simulink library "sllib"  (R2018a)
settings: Solver=VariableStepAuto  StartTime=0.0  StopTime=10.0  RelTol=1e-3
undefined symbols (not defined in the file or in its folder): In2, Mask_inport
libraries: simulink x12, simulink_extras x2
settings Model: Creator=zhoutinglin  LastModifiedBy=zhoutinglin

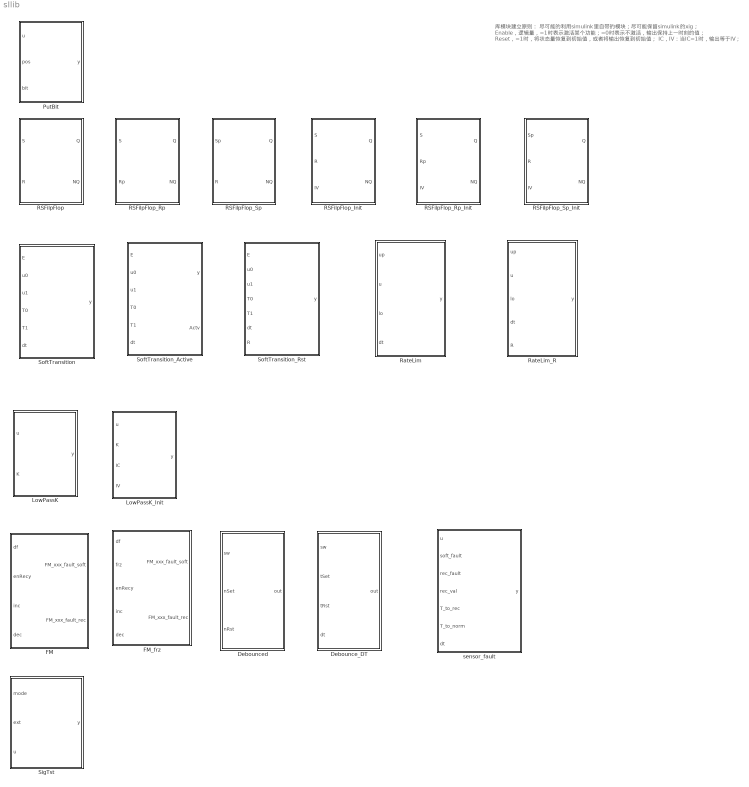
== system sllib ==
  note: 库模块建立原则：
      | 尽可能的利用simulink里自带的模块；尽可能保留simulink的xig；
      | Enable，逻辑量，=1时表示激活某个功能；=0时表示不激活，输出保持上一时刻的值；
      | Reset，=1时，将状态量恢复到初始值，或者将输出恢复到初始值；
      | IC，IV：当IC=1时，输出等于IV；
  Debounce_DT : Subsystem  mask(Debounce_DT){}
      mask help: 对一个开关形式的输入，当其状态改变时（从0变到1或者从1变到0），必须经过指定时间的确认之后再输出。
      mask Display:
      | color('blue');
      | plot([0.1,0.2,0.2,0.8,0.8,0.9],[0.26,0.26,0.46,0.46,0.26,0.26]);
      | plot([0.1,0.15,0.15,0.16,0.16,0.17,0.17,0.18,0.18,0.2,0.2,0.74,0.74,0.75,0.75,0.77,0.77,0.78,0.78,0.8,0.8,0.9],[0.55,0.55,0.75,0.75,0.55,0.55,0.75,0.75,0.55,0.55,0.75,0.75,0.55,0.55,0.75,0.75,0.55,0.55,0.75,0.75,0.55,0.55]);
  Debounced : Subsystem  mask(Debounced){}
      mask help: 对一个开关形式的输入，当其状态改变时（从0变到1或者从1变到0），必须经过指定次数的确认之后再输出。
      mask Display:
      | color('blue');
      | plot([0.1,0.2,0.2,0.8,0.8,0.9],[0.26,0.26,0.46,0.46,0.26,0.26]);
      | plot([0.1,0.15,0.15,0.16,0.16,0.17,0.17,0.18,0.18,0.2,0.2,0.74,0.74,0.75,0.75,0.77,0.77,0.78,0.78,0.8,0.8,0.9],[0.55,0.55,0.75,0.75,0.55,0.55,0.75,0.75,0.55,0.55,0.75,0.75,0.55,0.55,0.75,0.75,0.55,0.55,0.75,0.75,0.55,0.55]);
  FM : Subsystem  mask(FM){}
      mask help:
      | 输入df表示当前检测到的故障现象，等于1表示故障现象出现，等于0表示故障现象消失；
      | 输出soft故障等于输入df；
      | 输出rec故障等于soft故障经过Debounce后的状态。
  FM_frz : Subsystem  mask(FM_frz){}
      mask help:
      | 输入df表示当前检测到的故障现象，等于1表示故障现象出现，等于0表示故障现象消失；
      | 输出soft故障等于输入df；
      | 输出rec故障等于soft故障经过Debounce后的状态；
      | frz等于1后故障冻结，输出soft和rec的值不再变化，包括Debounce的计数器也不再变化。
  LowPassK : Subsystem  mask(LowPassK){}
      mask help: 低通滤波器
  LowPassK_Init : Subsystem  mask(LowPassK_Init){}
      mask help: 低通滤波器，带初始值。
  PutBit : Subsystem  mask(PutBit){}
      mask help: 给输入u在指定的位pos放入指定的值bit
  RSFilpFlop : Subsystem  mask(RSFlipFlop){}
      mask help: R和S都等于1时请参考真值表
  RSFilpFlop_Init : Subsystem  mask(RSFilpFlop_Init){}
      mask help:
      | R和S都等于1时请参考真值表;
      | 可以给Q赋初始值。
  RSFilpFlop_Rp : Subsystem  mask(RSFilpFlop_Rp){}
      mask help: R和S都等于1时的输出请参考真值表
  RSFilpFlop_Rp_Init : Subsystem  mask(RSFilpFlop_Rp_Init){}
      mask help:
      | R和S都等于1时请参考真值表;
      | 可以给Q赋初始值。
  RSFilpFlop_Sp : Subsystem  mask(RSFlipFlop_Sp){}
      mask help: R和S都等于1时的输出请参考真值表
  RSFilpFlop_Sp_Init : Subsystem  mask(RSFilpFlop_Sp_Init){}
      mask help:
      | R和S都等于1时请参考真值表;
      | 可以给Q赋初始值。
  RateLim : Subsystem  mask(RateLim){}
      mask help: 将输入信号u的变化速率限制在一定范围内。
  RateLim_R : Subsystem  mask(RateLim_R){}
      mask help: 将输入信号u的变化速率限制在一定范围内；当R置位时，输出y直接等于输入u。
  SigTst : Subsystem  mask(SigTst){}
      mask help:
      | 信号旁通功能，有3种模式：
      | mode=0时，直接输出u；
      | mode=1时，输出ext；
      | mode=2时，输出u+ext；
      mask Display:
      | color('white');
      | plot([0 0.01],[0 0.01]);
      | patch([0.65 0.67 0.67 0.65],[0.68 0.68 0.67 0.67]);
      | patch([0.65 0.67 0.67 0.65],[0.45 0.45 0.44 0.44]);
      | patch([0.65 0.67 0.67 0.65],[0.19 0.19 0.18 0.18]);
      | plot([0.18 0.65],[0.18 0.18]);
      | plot([0.18 0.65],[0.45 0.45]);
      | plot([0.24 0.4],[0.68 0.68]);
      | plot([0.57 0.65],[0.68 0.68]);
      | plot([0.4 0.57 0.57 0.4 0.4],[0.75 0.75 0.6 0.6 0.75]);
      | plot([0.49 0.49],[0.45 0.6]);
      | plot([0.45 0.52],[0.68 0.68]);
      | plot([0.49 0.49],[0.65 0.71]);
      | plot([0.24 0.24 0.26 0.26 0.24 0.24],[0.18 0.43 0.43 0.47 0.47 0.68]);
      | plot([0.25 0.85 0.85],[0.85 0.85 0.55]);
      | plot([0.7 0.8 0.95],[0.2 0.5 0.5]);
      | plot([0.83 0.85 0.88],[0.6 0.55 0.6])
  SoftTransition : Subsystem  mask(SoftTransition){}
      mask help: 当E改变时，输出缓慢过渡到u1或者u0.
  SoftTransition_Active : Subsystem  mask(SoftTransition_Active){}
      mask help:
      | 当E改变时，输出缓慢过渡到u1或者u0；
      | 输出Actv表示过渡是否已经结束。
  SoftTransition_Rst : Subsystem  mask(SoftTransition_Rst){}
      mask help:
      | 当E改变时，输出缓慢过渡到u1或者u0；
      | 当R置1时，直接输出目标值u1或者u0，不再过渡。
  sensor_fault : Subsystem  mask(sensor_fault){}
      mask help:
      | 当传感器无故障时，输出y直接等于输入u。
      | 当传感器有soft故障时，输出y等于其上一个时刻的值。
      | 当传感器故障被确认（rec）时，输出y过渡到rec_val；过渡时间为T_to_rec。
      | 当传感器从soft或rec状态恢复时，输出y经过时间T_to_norm过渡到u。

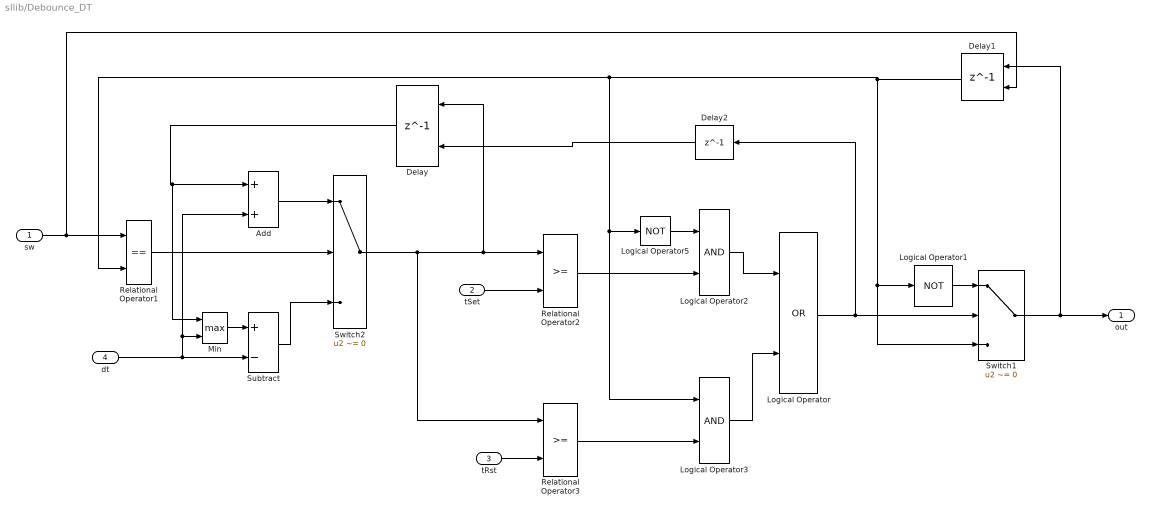
== system sllib/Debounce_DT ==
  sw : Inport  OutDataTypeStr=boolean
  tSet : Inport  Port=2
  tRst : Inport  Port=3
  dt : Inport  Port=4
  Add : Sum  SaturateOnIntegerOverflow=on  InputSameDT=on  OutDataTypeStr=Inherit: Same as first input
  Delay : Delay  DelayLength=1  ExternalReset=Rising
      settings: InputPortMap=u0,r5
  Delay1 : Delay  DelayLength=1  InitialConditionSource=Input port  InitialCondition=0
      settings: InputPortMap=u0,p4
  Delay2 : Delay  DelayLength=1  InitialCondition=0
  Logical Operator : Logic  Operator=OR  OutDataTypeStr=boolean
  Logical Operator1 : Logic  Operator=NOT  AllPortsSameDT=off  OutDataTypeStr=boolean
  Logical Operator2 : Logic  AllPortsSameDT=off  OutDataTypeStr=boolean
  Logical Operator3 : Logic  AllPortsSameDT=off  OutDataTypeStr=boolean
  Logical Operator5 : Logic  Operator=NOT  AllPortsSameDT=off  OutDataTypeStr=boolean
  Min : MinMax  Function=max  Inputs=2  ZeroCross=off  SaturateOnIntegerOverflow=on  InputSameDT=on
  Relational Operator1 : RelationalOperator  Operator===  OutDataTypeStr=boolean  ZeroCross=off  RndMeth=Simplest  InputSameDT=on
  Relational Operator2 : RelationalOperator  OutDataTypeStr=boolean  ZeroCross=off  RndMeth=Simplest  InputSameDT=on
  Relational Operator3 : RelationalOperator  OutDataTypeStr=boolean  ZeroCross=off  RndMeth=Simplest  InputSameDT=on
  Subtract : Sum  Inputs=+-  SaturateOnIntegerOverflow=on  InputSameDT=on
  Switch1 : Switch  Criteria=u2 ~= 0  ZeroCross=off
  Switch2 : Switch  Criteria=u2 ~= 0  ZeroCross=off  SaturateOnIntegerOverflow=on  InputSameDT=on
  out : Outport  OutDataTypeStr=boolean
  wires:
  Min/1 -> Subtract/1
  Delay2/1 -> Delay/2
  sw/1 -> Relational Operator1/1, Delay1/2
  Switch2/1 -> Relational Operator3/1, Delay/1, Relational Operator2/1
  Logical Operator/1 -> Switch1/2, Delay2/1
  Switch1/1 -> Delay1/1, out/1
  Delay/1 -> Add/1, Min/1
  Add/1 -> Switch2/1
  Relational Operator1/1 -> Switch2/2
  dt/1 -> Add/2, Min/2, Subtract/2
  Subtract/1 -> Switch2/3
  tSet/1 -> Relational Operator2/2
  tRst/1 -> Relational Operator3/2
  Logical Operator1/1 -> Switch1/1
  Relational Operator2/1 -> Logical Operator2/2
  Relational Operator3/1 -> Logical Operator3/2
  Delay1/1 -> Logical Operator3/1, Logical Operator5/1, Relational Operator1/2, Switch1/3, Logical Operator1/1
  Logical Operator2/1 -> Logical Operator/1
  Logical Operator3/1 -> Logical Operator/2
  Logical Operator5/1 -> Logical Operator2/1

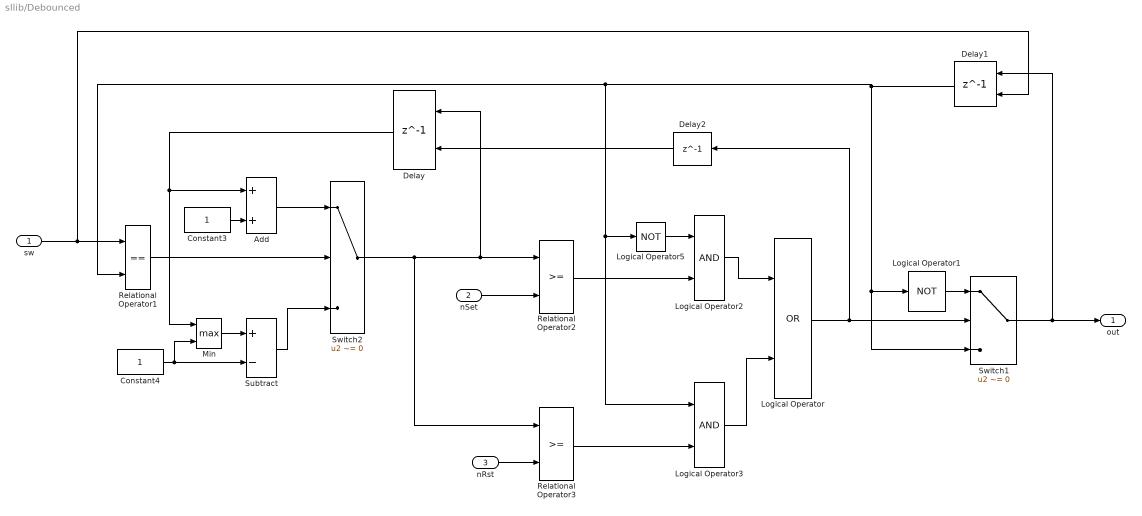
== system sllib/Debounced ==
  sw : Inport  OutDataTypeStr=boolean
  nSet : Inport  Port=2  OutDataTypeStr=uint16
  nRst : Inport  Port=3  OutDataTypeStr=uint16
  Add : Sum  SaturateOnIntegerOverflow=on  InputSameDT=on
  Constant3 : Constant  OutDataTypeStr=uint16
  Constant4 : Constant  OutDataTypeStr=uint16
  Delay : Delay  DelayLength=1  ExternalReset=Rising
      settings: InputPortMap=u0,r5
  Delay1 : Delay  DelayLength=1  InitialConditionSource=Input port
      settings: InputPortMap=u0,p4
  Delay2 : Delay  DelayLength=1  InitialCondition=0
  Logical Operator : Logic  Operator=OR  AllPortsSameDT=off  OutDataTypeStr=boolean
  Logical Operator1 : Logic  Operator=NOT  AllPortsSameDT=off  OutDataTypeStr=boolean
  Logical Operator2 : Logic  AllPortsSameDT=off  OutDataTypeStr=boolean
  Logical Operator3 : Logic  AllPortsSameDT=off  OutDataTypeStr=boolean
  Logical Operator5 : Logic  Operator=NOT  AllPortsSameDT=off  OutDataTypeStr=boolean
  Min : MinMax  Function=max  Inputs=2  ZeroCross=off  SaturateOnIntegerOverflow=on  InputSameDT=on
  Relational Operator1 : RelationalOperator  Operator===  OutDataTypeStr=boolean  ZeroCross=off  RndMeth=Simplest
  Relational Operator2 : RelationalOperator  OutDataTypeStr=boolean  ZeroCross=off  RndMeth=Simplest
  Relational Operator3 : RelationalOperator  OutDataTypeStr=boolean  ZeroCross=off  RndMeth=Simplest
  Subtract : Sum  Inputs=+-  SaturateOnIntegerOverflow=on  InputSameDT=on
  Switch1 : Switch  Criteria=u2 ~= 0  ZeroCross=off
  Switch2 : Switch  Criteria=u2 ~= 0  ZeroCross=off
  out : Outport  OutDataTypeStr=boolean
  wires:
  sw/1 -> Delay1/2, Relational Operator1/1
  Switch2/1 -> Relational Operator3/1, Delay/1, Relational Operator2/1
  Logical Operator/1 -> Switch1/2, Delay2/1
  Switch1/1 -> Delay1/1, out/1
  Delay/1 -> Min/1, Add/1
  Add/1 -> Switch2/1
  Relational Operator1/1 -> Switch2/2
  Constant3/1 -> Add/2
  Constant4/1 -> Subtract/2, Min/2
  Subtract/1 -> Switch2/3
  nSet/1 -> Relational Operator2/2
  nRst/1 -> Relational Operator3/2
  Logical Operator1/1 -> Switch1/1
  Relational Operator2/1 -> Logical Operator2/2
  Relational Operator3/1 -> Logical Operator3/2
  Delay1/1 -> Logical Operator3/1, Logical Operator5/1, Relational Operator1/2, Switch1/3, Logical Operator1/1
  Logical Operator2/1 -> Logical Operator/1
  Logical Operator3/1 -> Logical Operator/2
  Logical Operator5/1 -> Logical Operator2/1
  Delay2/1 -> Delay/2
  Min/1 -> Subtract/1

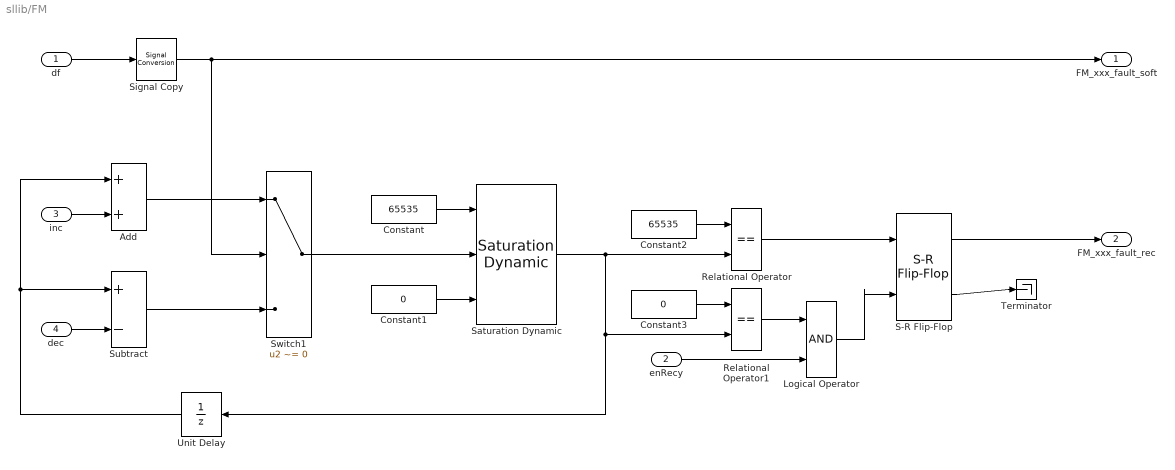
== system sllib/FM ==
  df : Inport  OutDataTypeStr=boolean
  enRecy : Inport  Port=2  OutDataTypeStr=boolean
  inc : Inport  LibraryBlock=Mask_inport/In2  Port=3  OutDataTypeStr=uint16
  dec : Inport  LibraryBlock=Mask_inport/In2  Port=4  OutDataTypeStr=uint16
  Add : Sum  SaturateOnIntegerOverflow=on  InputSameDT=on  OutDataTypeStr=Inherit: Same as first input
  Constant : Constant  Value=65535  OutDataTypeStr=uint16
  Constant1 : Constant  Value=0  OutDataTypeStr=uint16
  Constant2 : Constant  Value=65535  OutDataTypeStr=uint16
  Constant3 : Constant  Value=0  OutDataTypeStr=uint16
  Logical Operator : Logic  AllPortsSameDT=off  OutDataTypeStr=boolean
  Relational Operator : RelationalOperator  Operator===  OutDataTypeStr=boolean  ZeroCross=off  RndMeth=Simplest  InputSameDT=on
  Relational Operator1 : RelationalOperator  Operator===  OutDataTypeStr=boolean  ZeroCross=off  RndMeth=Simplest  InputSameDT=on
  S-R Flip-Flop : simulink_extras/Flip Flops/S-R Flip-Flop  initial_condition=0
      settings: AttributesFormatString=InitialValueQ=%<initial_condition>
  Saturation Dynamic : simulink/Discontinuities/Saturation Dynamic  OutMin=[]  OutMax=[]  OutDataTypeStr=Inherit: Same as second input  OutDataType=fixdt(1, 16)  OutScaling=2^-10  DoSatur=off
  Signal Copy : SignalConversion  OverrideOpt=off
  Subtract : Sum  Inputs=+-  SaturateOnIntegerOverflow=on  InputSameDT=on  OutDataTypeStr=Inherit: Same as first input
  Switch1 : Switch  Criteria=u2 ~= 0  ZeroCross=off  InputSameDT=on
  Terminator : Terminator
  Unit Delay : UnitDelay  SampleTime=-1
      settings: AttributesFormatString=InitialValue=%<InitialCondition>
  FM_xxx_fault_soft : Outport  OutDataTypeStr=boolean
  FM_xxx_fault_rec : Outport  Port=2  OutDataTypeStr=boolean
  wires:
  Signal Copy/1 -> FM_xxx_fault_soft/1, Switch1/2
  S-R Flip-Flop/1 -> FM_xxx_fault_rec/1
  S-R Flip-Flop/2 -> Terminator/1
  Logical Operator/1 -> S-R Flip-Flop/2
  Relational Operator/1 -> S-R Flip-Flop/1
  Relational Operator1/1 -> Logical Operator/1
  Constant3/1 -> Relational Operator1/1
  Saturation Dynamic/1 -> Relational Operator1/2, Unit Delay/1, Relational Operator/2
  Constant2/1 -> Relational Operator/1
  Constant1/1 -> Saturation Dynamic/3
  Constant/1 -> Saturation Dynamic/1
  Switch1/1 -> Saturation Dynamic/2
  Subtract/1 -> Switch1/3
  Add/1 -> Switch1/1
  Unit Delay/1 -> Add/1, Subtract/1
  inc/1 -> Add/2
  dec/1 -> Subtract/2
  enRecy/1 -> Logical Operator/2
  df/1 -> Signal Copy/1

== system sllib/FM_frz ==
  df : Inport  OutDataTypeStr=boolean
  frz : Inport  Port=2  OutDataTypeStr=boolean
  enRecy : Inport  Port=3  OutDataTypeStr=boolean
  inc : Inport  LibraryBlock=Mask_inport/In2  Port=4  OutDataTypeStr=uint16
  dec : Inport  LibraryBlock=Mask_inport/In2  Port=5  OutDataTypeStr=uint16
  rec : Subsystem
  soft : Subsystem
  FM_xxx_fault_soft : Outport  OutDataTypeStr=boolean
  FM_xxx_fault_rec : Outport  Port=2  OutDataTypeStr=boolean
  wires:
  inc/1 -> rec/4(inc)
  dec/1 -> rec/5(dec)
  soft/1(FM_xxx_fault_soft) -> FM_xxx_fault_soft/1
  rec/1(FM_xxx_fault_rec) -> FM_xxx_fault_rec/1
  df/1 -> rec/1(df), soft/1(df)
  frz/1 -> rec/2(frz), soft/2(frz)
  enRecy/1 -> rec/3(enRecy)

== system sllib/LowPassK ==
  u : Inport
  K : Inport  Port=2
  Delay : Delay  DelayLength=1  InitialConditionSource=Input port
      settings: InputPortMap=u0,p4
  Product : Product  RndMeth=Round  SaturateOnIntegerOverflow=on  OutDataTypeStr=Inherit: Same as first input
  Subtract1 : Sum  Inputs=+-  RndMeth=Round  SaturateOnIntegerOverflow=on  InputSameDT=on  OutDataTypeStr=Inherit: Same as first input
  Sum : Sum  Inputs=+|+  RndMeth=Round  SaturateOnIntegerOverflow=on  InputSameDT=on  OutDataTypeStr=Inherit: Same as first input
  y : Outport
  wires:
  u/1 -> Delay/2, Subtract1/1
  Delay/1 -> Sum/2, Subtract1/2
  Product/1 -> Sum/1
  Sum/1 -> Delay/1, y/1
  Subtract1/1 -> Product/1
  K/1 -> Product/2

== system sllib/LowPassK_Init ==
  u : Inport
  K : Inport  Port=2
  IC : Inport  Port=3  OutDataTypeStr=boolean
  IV : Inport  Port=4
  Delay : Delay  DelayLength=1  InitialConditionSource=Input port
      settings: InputPortMap=u0,p4
  Product : Product  RndMeth=Round  SaturateOnIntegerOverflow=on  OutDataTypeStr=Inherit: Same as first input
  Subtract1 : Sum  Inputs=+-  RndMeth=Round  SaturateOnIntegerOverflow=on  InputSameDT=on  OutDataTypeStr=Inherit: Same as first input
  Sum : Sum  Inputs=+|+  RndMeth=Round  SaturateOnIntegerOverflow=on  InputSameDT=on  OutDataTypeStr=Inherit: Same as first input
  Switch : Switch  Criteria=u2 ~= 0  RndMeth=Round  ZeroCross=off  InputSameDT=on
  y : Outport
  wires:
  Switch/1 -> Delay/1, y/1
  IC/1 -> Switch/2
  IV/1 -> Switch/1
  Subtract1/1 -> Product/1
  Delay/1 -> Sum/2, Subtract1/2
  u/1 -> Delay/2, Subtract1/1
  Sum/1 -> Switch/3
  Product/1 -> Sum/1
  K/1 -> Product/2

== system sllib/PutBit ==
  u : Inport
  pos : Inport  Port=2  OutDataTypeStr=uint8
  bit : Inport  Port=3  OutDataTypeStr=boolean
  Bitwise Operator : simulink/Logic and Bit Operations/Bitwise Operator  logicop=OR  UseBitMask=off  NumInputPorts=2  BitMask=bin2dec('11011001')  BitMaskRealWorld=Stored Integer
  Bitwise Operator1 : simulink/Logic and Bit Operations/Bitwise Operator  logicop=AND  UseBitMask=off  NumInputPorts=2  BitMask=bin2dec('11011001')  BitMaskRealWorld=Stored Integer
  Bitwise Operator2 : simulink/Logic and Bit Operations/Bitwise Operator  logicop=NOT  UseBitMask=off  BitMask=bin2dec('11011001')  BitMaskRealWorld=Stored Integer
  Constant2 : Constant  OutDataTypeStr=Inherit: Inherit via back propagation
  Data Type Duplicate : DataTypeDuplicate  NumInputPorts=3
  Shift Arithmetic : ArithShift  BitShiftNumberSource=Input port  BitShiftNumber=8  BitShiftDirection=Left
      settings: InputPortMap=u0,p1
  Switch : Switch  Criteria=u2 ~= 0  RndMeth=Round  ZeroCross=off  InputSameDT=on
  y : Outport
  wires:
  pos/1 -> Shift Arithmetic/2
  Constant2/1 -> Data Type Duplicate/2, Shift Arithmetic/1
  Shift Arithmetic/1 -> Bitwise Operator2/1, Bitwise Operator/2
  bit/1 -> Switch/2
  Bitwise Operator/1 -> Switch/1
  u/1 -> Data Type Duplicate/1, Bitwise Operator1/1, Bitwise Operator/1
  Bitwise Operator2/1 -> Bitwise Operator1/2
  Bitwise Operator1/1 -> Switch/3
  Switch/1 -> Data Type Duplicate/3, y/1

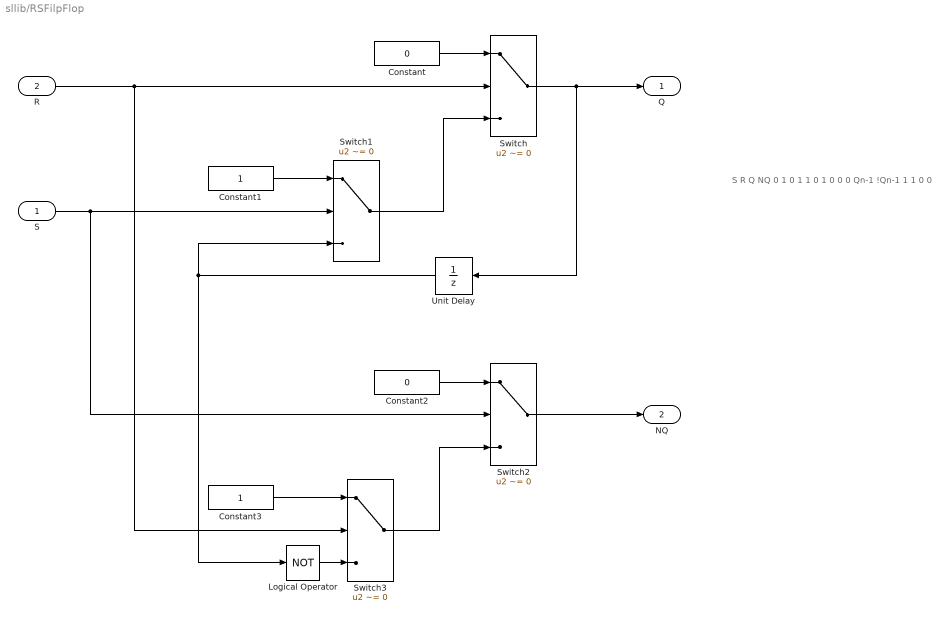
== system sllib/RSFilpFlop ==
  note: S
      | R
      | Q
      | NQ
      |
      | 0
      | 1
      | 0
      | 1
      |
      | 1
      | 0
      | 1
      | 0
      |
      | 0
      | 0
      | Qn-1
      | !Qn-1
      |
      | 1
      | 1
      | 0
      | 0
  S : Inport  OutDataTypeStr=boolean
  R : Inport  Port=2  OutDataTypeStr=boolean
  Constant : Constant  Value=0  OutDataTypeStr=boolean
  Constant1 : Constant  OutDataTypeStr=boolean
  Constant2 : Constant  Value=0  OutDataTypeStr=boolean
  Constant3 : Constant  OutDataTypeStr=boolean
  Logical Operator : Logic  Operator=NOT  AllPortsSameDT=off  OutDataTypeStr=boolean
  Switch{,1..3} (4 alike) : Switch  Criteria=u2 ~= 0  ZeroCross=off
  Unit Delay : UnitDelay  SampleTime=-1
      settings: AttributesFormatString=InitialValue=%<InitialCondition>
  Q : Outport  OutDataTypeStr=boolean
  NQ : Outport  Port=2  OutDataTypeStr=boolean
  wires:
  R/1 -> Switch3/2, Switch/2
  Constant/1 -> Switch/1
  Switch/1 -> Unit Delay/1, Q/1
  S/1 -> Switch2/2, Switch1/2
  Constant1/1 -> Switch1/1
  Switch1/1 -> Switch/3
  Unit Delay/1 -> Switch1/3, Logical Operator/1
  Switch2/1 -> NQ/1
  Constant2/1 -> Switch2/1
  Switch3/1 -> Switch2/3
  Constant3/1 -> Switch3/1
  Logical Operator/1 -> Switch3/3

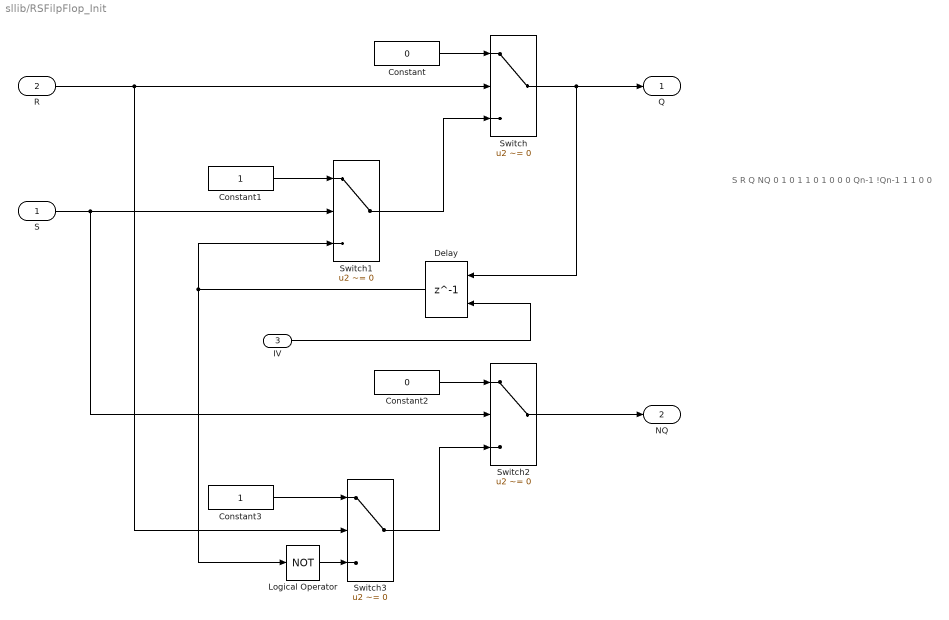
== system sllib/RSFilpFlop_Init ==
  note: S
      | R
      | Q
      | NQ
      |
      | 0
      | 1
      | 0
      | 1
      |
      | 1
      | 0
      | 1
      | 0
      |
      | 0
      | 0
      | Qn-1
      | !Qn-1
      |
      | 1
      | 1
      | 0
      | 0
  S : Inport  OutDataTypeStr=boolean
  R : Inport  Port=2  OutDataTypeStr=boolean
  IV : Inport  Port=3
  Constant : Constant  Value=0  OutDataTypeStr=boolean
  Constant1 : Constant  OutDataTypeStr=boolean
  Constant2 : Constant  Value=0  OutDataTypeStr=boolean
  Constant3 : Constant  OutDataTypeStr=boolean
  Delay : Delay  DelayLength=1  InitialConditionSource=Input port
      settings: InputPortMap=u0,p4
  Logical Operator : Logic  Operator=NOT  AllPortsSameDT=off  OutDataTypeStr=boolean
  Switch{,1..3} (4 alike) : Switch  Criteria=u2 ~= 0  ZeroCross=off
  Q : Outport  OutDataTypeStr=boolean
  NQ : Outport  Port=2  OutDataTypeStr=boolean
  wires:
  R/1 -> Switch3/2, Switch/2
  Constant/1 -> Switch/1
  Switch/1 -> Delay/1, Q/1
  S/1 -> Switch2/2, Switch1/2
  Constant1/1 -> Switch1/1
  Switch1/1 -> Switch/3
  Delay/1 -> Switch1/3, Logical Operator/1
  Switch2/1 -> NQ/1
  Constant2/1 -> Switch2/1
  Switch3/1 -> Switch2/3
  Constant3/1 -> Switch3/1
  Logical Operator/1 -> Switch3/3
  IV/1 -> Delay/2

== system sllib/RSFilpFlop_Rp ==
  note: S
      | R
      | Q
      | NQ
      |
      | 0
      | 1
      | 0
      | 1
      |
      | 1
      | 0
      | 1
      | 0
      |
      | 0
      | 0
      | Qn-1
      | !Qn-1
      |
      | 1
      | 1
      | 0
      | 1
  S : Inport  OutDataTypeStr=boolean
  Rp : Inport  Port=2  OutDataTypeStr=boolean
  Constant : Constant  Value=0  OutDataTypeStr=boolean
  Constant1 : Constant  OutDataTypeStr=boolean
  Logical Operator : Logic  Operator=NOT  AllPortsSameDT=off  OutDataTypeStr=boolean
  Switch : Switch  Criteria=u2 ~= 0  ZeroCross=off
  Switch1 : Switch  Criteria=u2 ~= 0  ZeroCross=off
  Unit Delay : UnitDelay  SampleTime=-1
      settings: AttributesFormatString=InitialValue=%<InitialCondition>
  Q : Outport  OutDataTypeStr=boolean
  NQ : Outport  Port=2  OutDataTypeStr=boolean
  wires:
  Rp/1 -> Switch/2
  Constant/1 -> Switch/1
  Switch/1 -> Logical Operator/1, Unit Delay/1, Q/1
  S/1 -> Switch1/2
  Constant1/1 -> Switch1/1
  Switch1/1 -> Switch/3
  Unit Delay/1 -> Switch1/3
  Logical Operator/1 -> NQ/1

== system sllib/RSFilpFlop_Rp_Init ==
  note: S
      | R
      | Q
      | NQ
      |
      | 0
      | 1
      | 0
      | 1
      |
      | 1
      | 0
      | 1
      | 0
      |
      | 0
      | 0
      | Qn-1
      | !Qn-1
      |
      | 1
      | 1
      | 0
      | 1
  S : Inport  OutDataTypeStr=boolean
  Rp : Inport  Port=2  OutDataTypeStr=boolean
  IV : Inport  Port=3
  Constant : Constant  Value=0  OutDataTypeStr=boolean
  Constant1 : Constant  OutDataTypeStr=boolean
  Delay : Delay  DelayLength=1  InitialConditionSource=Input port
      settings: InputPortMap=u0,p4
  Logical Operator : Logic  Operator=NOT  AllPortsSameDT=off  OutDataTypeStr=boolean
  Switch : Switch  Criteria=u2 ~= 0  ZeroCross=off
  Switch1 : Switch  Criteria=u2 ~= 0  ZeroCross=off
  Q : Outport  OutDataTypeStr=boolean
  NQ : Outport  Port=2  OutDataTypeStr=boolean
  wires:
  Rp/1 -> Switch/2
  Constant/1 -> Switch/1
  Switch/1 -> Delay/1, Logical Operator/1, Q/1
  S/1 -> Switch1/2
  Constant1/1 -> Switch1/1
  Switch1/1 -> Switch/3
  Delay/1 -> Switch1/3
  Logical Operator/1 -> NQ/1
  IV/1 -> Delay/2

== system sllib/RSFilpFlop_Sp ==
  note: S
      | R
      | Q
      | NQ
      |
      | 0
      | 1
      | 0
      | 1
      |
      | 1
      | 0
      | 1
      | 0
      |
      | 0
      | 0
      | Qn-1
      | !Qn-1
      |
      | 1
      | 1
      | 1
      | 0
  Sp : Inport  OutDataTypeStr=boolean
  R : Inport  Port=2  OutDataTypeStr=boolean
  Constant : Constant  OutDataTypeStr=boolean
  Constant1 : Constant  Value=0  OutDataTypeStr=boolean
  Logical Operator : Logic  Operator=NOT  AllPortsSameDT=off  OutDataTypeStr=boolean
  Switch : Switch  Criteria=u2 ~= 0  ZeroCross=off
  Switch1 : Switch  Criteria=u2 ~= 0  ZeroCross=off
  Unit Delay : UnitDelay  SampleTime=-1
      settings: AttributesFormatString=InitialValue=%<InitialCondition>
  Q : Outport  OutDataTypeStr=boolean
  NQ : Outport  Port=2  OutDataTypeStr=boolean
  wires:
  Constant/1 -> Switch/1
  Switch/1 -> Logical Operator/1, Unit Delay/1, Q/1
  Constant1/1 -> Switch1/1
  Switch1/1 -> Switch/3
  Unit Delay/1 -> Switch1/3
  Logical Operator/1 -> NQ/1
  Sp/1 -> Switch/2
  R/1 -> Switch1/2

== system sllib/RSFilpFlop_Sp_Init ==
  note: S
      | R
      | Q
      | NQ
      |
      | 0
      | 1
      | 0
      | 1
      |
      | 1
      | 0
      | 1
      | 0
      |
      | 0
      | 0
      | Qn-1
      | !Qn-1
      |
      | 1
      | 1
      | 1
      | 0
  Sp : Inport  OutDataTypeStr=boolean
  R : Inport  Port=2  OutDataTypeStr=boolean
  IV : Inport  Port=3
  Constant : Constant  OutDataTypeStr=boolean
  Constant1 : Constant  Value=0  OutDataTypeStr=boolean
  Delay : Delay  DelayLength=1  InitialConditionSource=Input port
      settings: InputPortMap=u0,p4
  Logical Operator : Logic  Operator=NOT  AllPortsSameDT=off  OutDataTypeStr=boolean
  Switch : Switch  Criteria=u2 ~= 0  ZeroCross=off
  Switch1 : Switch  Criteria=u2 ~= 0  ZeroCross=off
  Q : Outport  OutDataTypeStr=boolean
  NQ : Outport  Port=2  OutDataTypeStr=boolean
  wires:
  Constant/1 -> Switch/1
  Switch/1 -> Delay/1, Logical Operator/1, Q/1
  Constant1/1 -> Switch1/1
  Switch1/1 -> Switch/3
  Delay/1 -> Switch1/3
  Logical Operator/1 -> NQ/1
  Sp/1 -> Switch/2
  R/1 -> Switch1/2
  IV/1 -> Delay/2

== system sllib/RateLim ==
  up : Inport
  u : Inport  Port=2
  lo : Inport  Port=3
  dt : Inport  Port=4
  Add : Sum  SaturateOnIntegerOverflow=on  InputSameDT=on  OutDataTypeStr=Inherit: Same as first input
  Data Type Duplicate : DataTypeDuplicate  NumInputPorts=3
  Delay : Delay  DelayLength=1  InitialConditionSource=Input port
      settings: InputPortMap=u0,p4
  Product : Product  OutDataTypeStr=Inherit: Same as first input
  Product1 : Product  SaturateOnIntegerOverflow=on  OutDataTypeStr=Inherit: Same as first input
  Saturation Dynamic : simulink/Discontinuities/Saturation Dynamic  OutMin=[]  OutMax=[]  OutDataTypeStr=Inherit: Same as second input  OutDataType=fixdt(1, 16)  OutScaling=2^-10  DoSatur=off
  Subtract : Sum  Inputs=+-  SaturateOnIntegerOverflow=on  InputSameDT=on  OutDataTypeStr=Inherit: Same as first input
  y : Outport
  wires:
  Saturation Dynamic/1 -> Add/1
  Add/1 -> y/1, Delay/1
  Delay/1 -> Subtract/2, Add/2
  u/1 -> Delay/2, Data Type Duplicate/1, Subtract/1
  Product/1 -> Saturation Dynamic/3
  Product1/1 -> Saturation Dynamic/1
  Subtract/1 -> Saturation Dynamic/2
  lo/1 -> Product/1, Data Type Duplicate/2
  up/1 -> Data Type Duplicate/3, Product1/1
  dt/1 -> Product1/2, Product/2

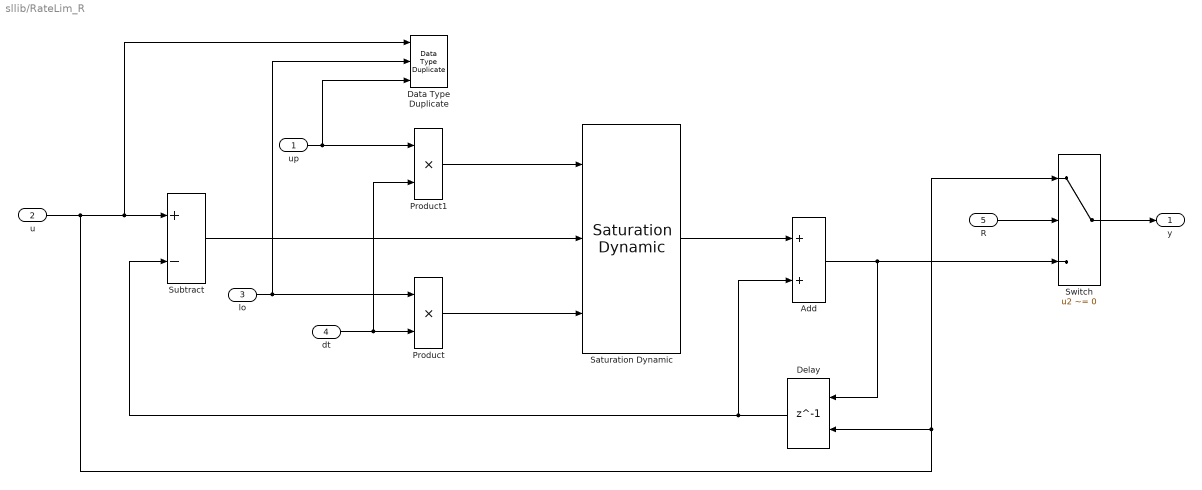
== system sllib/RateLim_R ==
  up : Inport
  u : Inport  Port=2
  lo : Inport  Port=3
  dt : Inport  Port=4
  R : Inport  Port=5  OutDataTypeStr=boolean
  Add : Sum  SaturateOnIntegerOverflow=on  InputSameDT=on  OutDataTypeStr=Inherit: Same as first input
  Data Type Duplicate : DataTypeDuplicate  NumInputPorts=3
  Delay : Delay  DelayLength=1  InitialConditionSource=Input port
      settings: InputPortMap=u0,p4
  Product : Product  OutDataTypeStr=Inherit: Same as first input
  Product1 : Product  SaturateOnIntegerOverflow=on  OutDataTypeStr=Inherit: Same as first input
  Saturation Dynamic : simulink/Discontinuities/Saturation Dynamic  OutMin=[]  OutMax=[]  OutDataTypeStr=Inherit: Same as second input  OutDataType=fixdt(1, 16)  OutScaling=2^-10  DoSatur=off
  Subtract : Sum  Inputs=+-  SaturateOnIntegerOverflow=on  InputSameDT=on  OutDataTypeStr=Inherit: Same as first input
  Switch : Switch  Criteria=u2 ~= 0  ZeroCross=off  InputSameDT=on
  y : Outport
  wires:
  Saturation Dynamic/1 -> Add/1
  Add/1 -> Switch/3, Delay/1
  Delay/1 -> Subtract/2, Add/2
  Product/1 -> Saturation Dynamic/3
  Product1/1 -> Saturation Dynamic/1
  Subtract/1 -> Saturation Dynamic/2
  lo/1 -> Product/1, Data Type Duplicate/2
  up/1 -> Data Type Duplicate/3, Product1/1
  dt/1 -> Product1/2, Product/2
  R/1 -> Switch/2
  Switch/1 -> y/1
  u/1 -> Switch/1, Delay/2, Data Type Duplicate/1, Subtract/1

== system sllib/SigTst ==
  mode : Inport
  ext : Inport  Port=2
  u : Inport  Port=3
  Add : Sum  SaturateOnIntegerOverflow=on  InputSameDT=on
  Constant : Constant  Value=2  OutDataTypeStr=Inherit: Inherit via back propagation
  Constant1 : Constant  OutDataTypeStr=Inherit: Inherit via back propagation
  Relational Operator : RelationalOperator  Operator===  OutDataTypeStr=boolean  ZeroCross=off  RndMeth=Simplest  InputSameDT=on
  Relational Operator1 : RelationalOperator  Operator===  OutDataTypeStr=boolean  ZeroCross=off  RndMeth=Simplest  InputSameDT=on
  Switch : Switch  Criteria=u2 ~= 0  ZeroCross=off  InputSameDT=on
  Switch1 : Switch  Criteria=u2 ~= 0  ZeroCross=off  InputSameDT=on
  y : Outport
  wires:
  mode/1 -> Relational Operator/1, Relational Operator1/1
  Constant/1 -> Relational Operator/2
  Constant1/1 -> Relational Operator1/2
  Relational Operator/1 -> Switch1/2
  u/1 -> Add/1, Switch/3
  Switch1/1 -> y/1
  Relational Operator1/1 -> Switch/2
  ext/1 -> Add/2, Switch/1
  Switch/1 -> Switch1/3
  Add/1 -> Switch1/1

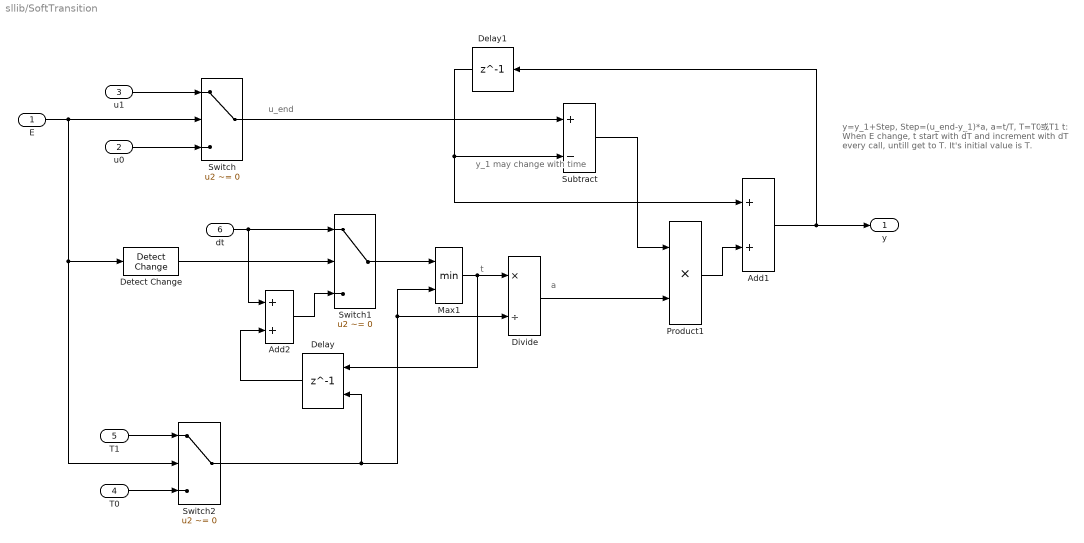
== system sllib/SoftTransition ==
  note: y_1 may change
      |  with time
  note: t
  note: a
  note: u_end
  note: y=y_1+Step, Step=(u_end-y_1)*a, a=t/T, T=T0或T1
      | t: When E change, t start with dT and increment with dT every call, untill get to T. It's initial value is T.
  E : Inport
  u0 : Inport  Port=2
  u1 : Inport  Port=3
  T0 : Inport  Port=4
  T1 : Inport  Port=5
  dt : Inport  Port=6
  Add1 : Sum  RndMeth=Round  SaturateOnIntegerOverflow=on  InputSameDT=on  OutDataTypeStr=Inherit: Same as first input
  Add2 : Sum  RndMeth=Round  SaturateOnIntegerOverflow=on  InputSameDT=on  OutDataTypeStr=Inherit: Same as first input
  Delay : Delay  DelayLength=1  InitialConditionSource=Input port
      settings: InputPortMap=u0,p4
  Delay1 : Delay  DelayLength=1
  Detect Change : simulink/Logic and Bit Operations/Detect Change  vinit=0  OutDataTypeStr=boolean
  Divide : Product  Inputs=*/  OutDataTypeStr=fixdt(1,16,2^-14,0)  RndMeth=Round  SaturateOnIntegerOverflow=on  InputSameDT=on
  Max1 : MinMax  Inputs=2  ZeroCross=off  InputSameDT=on
  Product1 : Product  RndMeth=Round  SaturateOnIntegerOverflow=on  OutDataTypeStr=Inherit: Same as first input
  Subtract : Sum  Inputs=+-  RndMeth=Round  SaturateOnIntegerOverflow=on  InputSameDT=on  OutDataTypeStr=Inherit: Same as first input
  Switch : Switch  Criteria=u2 ~= 0  ZeroCross=off  InputSameDT=on
  Switch1 : Switch  Criteria=u2 ~= 0  ZeroCross=off  InputSameDT=on
  Switch2 : Switch  Criteria=u2 ~= 0  ZeroCross=off  InputSameDT=on
  y : Outport
  wires:
  E/1 -> Detect Change/1, Switch2/2, Switch/2
  u1/1 -> Switch/1
  u0/1 -> Switch/3
  Switch2/1 -> Divide/2, Max1/2, Delay/2
  Delay/1 -> Add2/2
  T1/1 -> Switch2/1
  T0/1 -> Switch2/3
  Max1/1 -> Delay/1, Divide/1
  Divide/1 -> Product1/2
  Add1/1 -> y/1, Delay1/1
  Product1/1 -> Add1/2
  Delay1/1 -> Subtract/2, Add1/1
  Switch/1 -> Subtract/1
  Subtract/1 -> Product1/1
  Add2/1 -> Switch1/3
  Detect Change/1 -> Switch1/2
  dt/1 -> Add2/1, Switch1/1
  Switch1/1 -> Max1/1

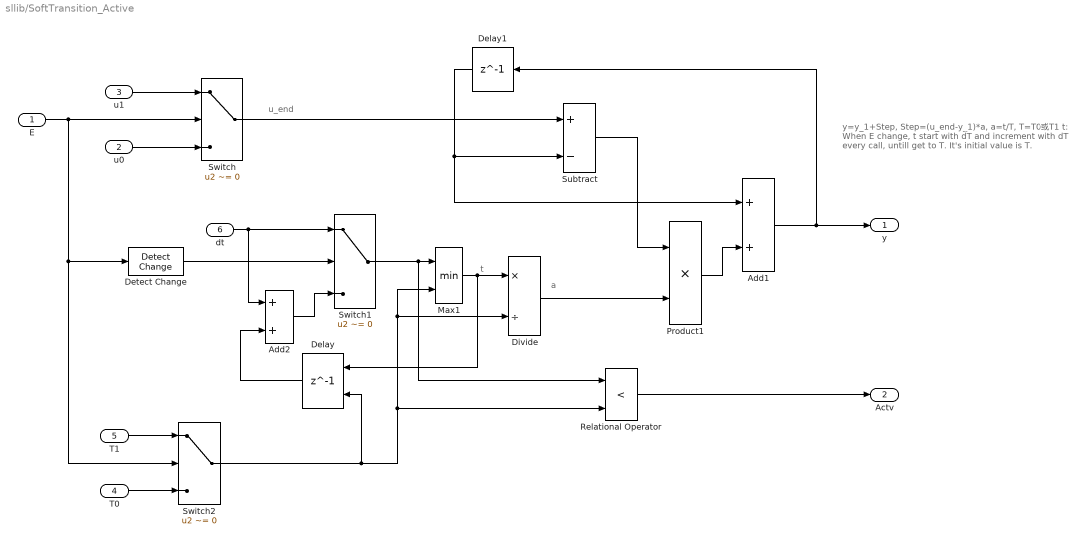
== system sllib/SoftTransition_Active ==
  note: t
  note: a
  note: u_end
  note: y=y_1+Step, Step=(u_end-y_1)*a, a=t/T, T=T0或T1
      | t: When E change, t start with dT and increment with dT every call, untill get to T. It's initial value is T.
  E : Inport
  u0 : Inport  Port=2
  u1 : Inport  Port=3
  T0 : Inport  Port=4
  T1 : Inport  Port=5
  dt : Inport  Port=6
  Add1 : Sum  RndMeth=Round  SaturateOnIntegerOverflow=on  InputSameDT=on  OutDataTypeStr=Inherit: Same as first input
  Add2 : Sum  RndMeth=Round  SaturateOnIntegerOverflow=on  InputSameDT=on  OutDataTypeStr=Inherit: Same as first input
  Delay : Delay  DelayLength=1  InitialConditionSource=Input port
      settings: InputPortMap=u0,p4
  Delay1 : Delay  DelayLength=1
  Detect Change : simulink/Logic and Bit Operations/Detect Change  vinit=0  OutDataTypeStr=boolean
  Divide : Product  Inputs=*/  OutDataTypeStr=fixdt(1,16,2^-14,0)  RndMeth=Round  SaturateOnIntegerOverflow=on  InputSameDT=on
  Max1 : MinMax  Inputs=2  ZeroCross=off  InputSameDT=on
  Product1 : Product  RndMeth=Round  SaturateOnIntegerOverflow=on  OutDataTypeStr=Inherit: Same as first input
  Relational Operator : RelationalOperator  Operator=<  OutDataTypeStr=boolean  ZeroCross=off  RndMeth=Simplest  InputSameDT=on
  Subtract : Sum  Inputs=+-  RndMeth=Round  SaturateOnIntegerOverflow=on  InputSameDT=on  OutDataTypeStr=Inherit: Same as first input
  Switch : Switch  Criteria=u2 ~= 0  ZeroCross=off  InputSameDT=on
  Switch1 : Switch  Criteria=u2 ~= 0  ZeroCross=off  InputSameDT=on
  Switch2 : Switch  Criteria=u2 ~= 0  ZeroCross=off  InputSameDT=on
  y : Outport
  Actv : Outport  Port=2
  wires:
  E/1 -> Detect Change/1, Switch2/2, Switch/2
  u1/1 -> Switch/1
  u0/1 -> Switch/3
  Delay/1 -> Add2/2
  T1/1 -> Switch2/1
  T0/1 -> Switch2/3
  Max1/1 -> Delay/1, Divide/1
  Divide/1 -> Product1/2
  Add1/1 -> y/1, Delay1/1
  Product1/1 -> Add1/2
  Delay1/1 -> Subtract/2, Add1/1
  Switch/1 -> Subtract/1
  Subtract/1 -> Product1/1
  Add2/1 -> Switch1/3
  Detect Change/1 -> Switch1/2
  dt/1 -> Add2/1, Switch1/1
  Switch1/1 -> Relational Operator/1, Max1/1
  Switch2/1 -> Relational Operator/2, Divide/2, Max1/2, Delay/2
  Relational Operator/1 -> Actv/1

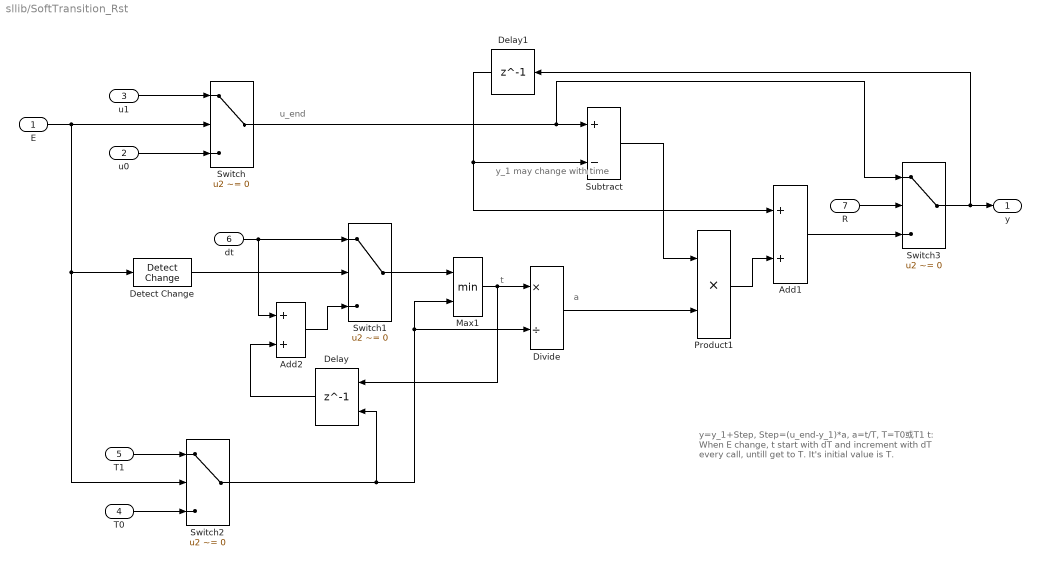
== system sllib/SoftTransition_Rst ==
  note: y_1 may change
      |  with time
  note: t
  note: a
  note: u_end
  note: y=y_1+Step, Step=(u_end-y_1)*a, a=t/T, T=T0或T1
      | t: When E change, t start with dT and increment with dT every call, untill get to T. It's initial value is T.
  E : Inport
  u0 : Inport  Port=2
  u1 : Inport  Port=3
  T0 : Inport  Port=4
  T1 : Inport  Port=5
  dt : Inport  Port=6
  R : Inport  Port=7  OutDataTypeStr=boolean
  Add1 : Sum  RndMeth=Round  SaturateOnIntegerOverflow=on  InputSameDT=on  OutDataTypeStr=Inherit: Same as first input
  Add2 : Sum  RndMeth=Round  SaturateOnIntegerOverflow=on  InputSameDT=on  OutDataTypeStr=Inherit: Same as first input
  Delay : Delay  DelayLength=1  InitialConditionSource=Input port
      settings: InputPortMap=u0,p4
  Delay1 : Delay  DelayLength=1
  Detect Change : simulink/Logic and Bit Operations/Detect Change  vinit=0  OutDataTypeStr=boolean
  Divide : Product  Inputs=*/  OutDataTypeStr=fixdt(1,16,2^-14,0)  RndMeth=Round  SaturateOnIntegerOverflow=on  InputSameDT=on
  Max1 : MinMax  Inputs=2  ZeroCross=off  InputSameDT=on
  Product1 : Product  RndMeth=Round  SaturateOnIntegerOverflow=on  OutDataTypeStr=Inherit: Same as first input
  Subtract : Sum  Inputs=+-  RndMeth=Round  SaturateOnIntegerOverflow=on  InputSameDT=on  OutDataTypeStr=Inherit: Same as first input
  Switch{,1..3} (4 alike) : Switch  Criteria=u2 ~= 0  ZeroCross=off  InputSameDT=on
  y : Outport
  wires:
  E/1 -> Detect Change/1, Switch2/2, Switch/2
  u1/1 -> Switch/1
  u0/1 -> Switch/3
  Switch2/1 -> Divide/2, Max1/2, Delay/2
  Delay/1 -> Add2/2
  T1/1 -> Switch2/1
  T0/1 -> Switch2/3
  Max1/1 -> Delay/1, Divide/1
  Divide/1 -> Product1/2
  Product1/1 -> Add1/2
  Delay1/1 -> Subtract/2, Add1/1
  Switch/1 -> Subtract/1, Switch3/1
  Subtract/1 -> Product1/1
  Add2/1 -> Switch1/3
  Detect Change/1 -> Switch1/2
  dt/1 -> Add2/1, Switch1/1
  Switch1/1 -> Max1/1
  R/1 -> Switch3/2
  Add1/1 -> Switch3/3
  Switch3/1 -> Delay1/1, y/1

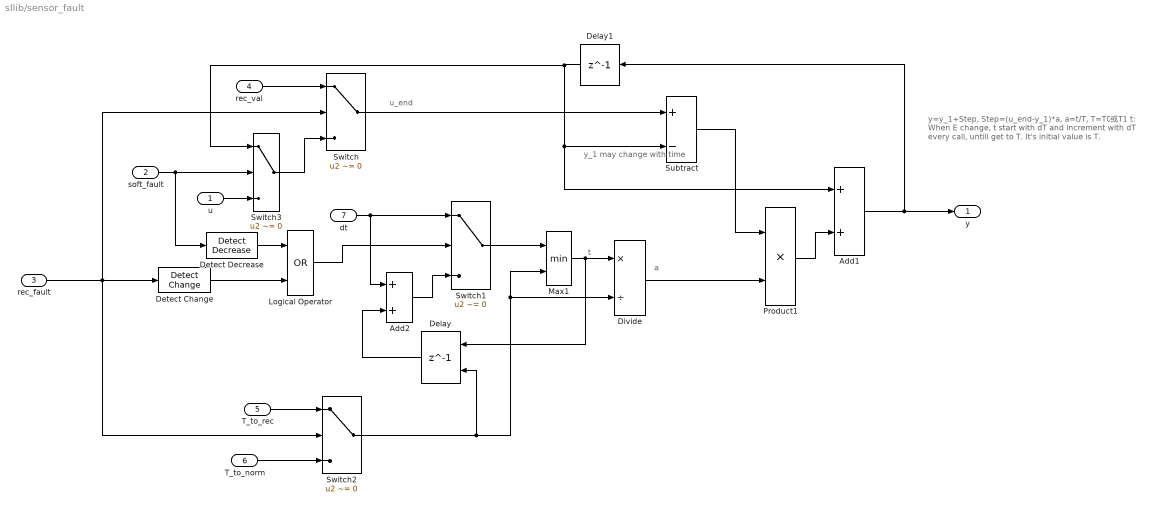
== system sllib/sensor_fault ==
  note: y=y_1+Step, Step=(u_end-y_1)*a, a=t/T, T=T0或T1
      | t: When E change, t start with dT and increment with dT every call, untill get to T. It's initial value is T.
  note: u_end
  note: a
  note: t
  note: y_1 may change
      |  with time
  u : Inport
  soft_fault : Inport  Port=2  OutDataTypeStr=boolean
  rec_fault : Inport  Port=3  OutDataTypeStr=boolean
  rec_val : Inport  Port=4
  T_to_rec : Inport  Port=5
  T_to_norm : Inport  Port=6
  dt : Inport  Port=7
  Add1 : Sum  RndMeth=Round  SaturateOnIntegerOverflow=on  InputSameDT=on  OutDataTypeStr=Inherit: Same as first input
  Add2 : Sum  RndMeth=Round  SaturateOnIntegerOverflow=on  InputSameDT=on  OutDataTypeStr=Inherit: Same as first input
  Delay : Delay  DelayLength=1  InitialConditionSource=Input port
      settings: InputPortMap=u0,p4
  Delay1 : Delay  DelayLength=1
  Detect Change : simulink/Logic and Bit Operations/Detect Change  vinit=0  OutDataTypeStr=boolean
  Detect Decrease : simulink/Logic and Bit Operations/Detect Decrease  vinit=0.0  OutDataTypeStr=boolean
  Divide : Product  Inputs=*/  OutDataTypeStr=fixdt(1,16,2^-14,0)  RndMeth=Round  SaturateOnIntegerOverflow=on  InputSameDT=on
  Logical Operator : Logic  Operator=OR  OutDataTypeStr=boolean
  Max1 : MinMax  Inputs=2  ZeroCross=off  InputSameDT=on
  Product1 : Product  RndMeth=Round  SaturateOnIntegerOverflow=on  OutDataTypeStr=Inherit: Same as first input
  Subtract : Sum  Inputs=+-  RndMeth=Round  SaturateOnIntegerOverflow=on  InputSameDT=on  OutDataTypeStr=Inherit: Same as first input
  Switch{,1..3} (4 alike) : Switch  Criteria=u2 ~= 0  ZeroCross=off  InputSameDT=on
  y : Outport
  wires:
  Logical Operator/1 -> Switch1/2
  Detect Change/1 -> Logical Operator/2
  Detect Decrease/1 -> Logical Operator/1
  Switch3/1 -> Switch/3
  rec_val/1 -> Switch/1
  soft_fault/1 -> Switch3/2, Detect Decrease/1
  u/1 -> Switch3/3
  rec_fault/1 -> Detect Change/1, Switch2/2, Switch/2
  Switch1/1 -> Max1/1
  dt/1 -> Switch1/1, Add2/1
  Add2/1 -> Switch1/3
  Subtract/1 -> Product1/1
  Switch/1 -> Subtract/1
  Delay1/1 -> Add1/1, Subtract/2, Switch3/1
  Product1/1 -> Add1/2
  Add1/1 -> Delay1/1, y/1
  Divide/1 -> Product1/2
  Max1/1 -> Divide/1, Delay/1
  T_to_norm/1 -> Switch2/3
  T_to_rec/1 -> Switch2/1
  Delay/1 -> Add2/2
  Switch2/1 -> Delay/2, Max1/2, Divide/2

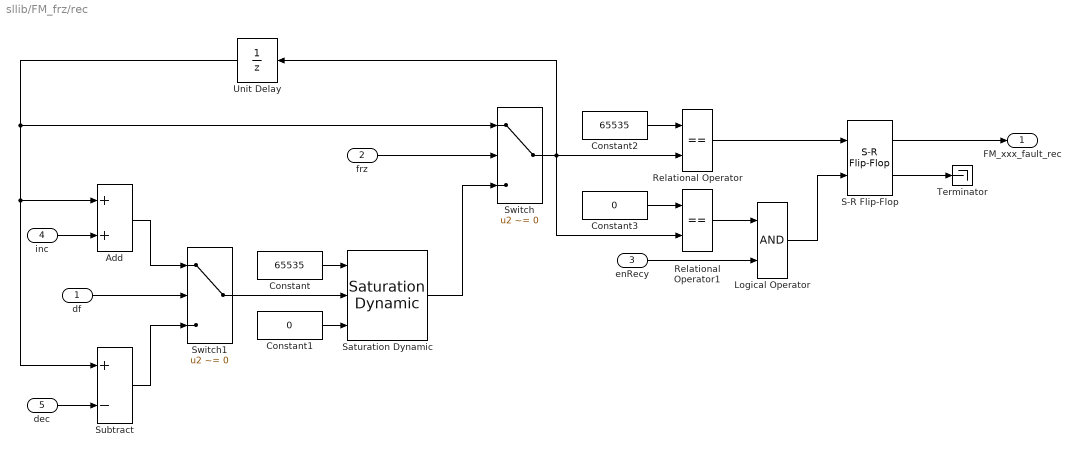
== system sllib/FM_frz/rec ==
  df : Inport  OutDataTypeStr=boolean
  frz : Inport  Port=2  OutDataTypeStr=boolean
  enRecy : Inport  Port=3  OutDataTypeStr=boolean
  inc : Inport  LibraryBlock=Mask_inport/In2  Port=4  OutDataTypeStr=uint16
  dec : Inport  LibraryBlock=Mask_inport/In2  Port=5  OutDataTypeStr=uint16
  Add : Sum  SaturateOnIntegerOverflow=on  InputSameDT=on  OutDataTypeStr=Inherit: Same as first input
  Constant : Constant  Value=65535  OutDataTypeStr=uint16
  Constant1 : Constant  Value=0  OutDataTypeStr=uint16
  Constant2 : Constant  Value=65535  OutDataTypeStr=uint16
  Constant3 : Constant  Value=0  OutDataTypeStr=uint16
  Logical Operator : Logic  AllPortsSameDT=off  OutDataTypeStr=boolean
  Relational Operator : RelationalOperator  Operator===  OutDataTypeStr=boolean  ZeroCross=off  RndMeth=Simplest  InputSameDT=on
  Relational Operator1 : RelationalOperator  Operator===  OutDataTypeStr=boolean  ZeroCross=off  RndMeth=Simplest  InputSameDT=on
  S-R Flip-Flop : simulink_extras/Flip Flops/S-R Flip-Flop  initial_condition=0
      settings: AttributesFormatString=InitialValueQ=%<initial_condition>
  Saturation Dynamic : simulink/Discontinuities/Saturation Dynamic  OutMin=[]  OutMax=[]  OutDataTypeStr=Inherit: Same as second input  OutDataType=fixdt(1, 16)  OutScaling=2^-10  DoSatur=off
  Subtract : Sum  Inputs=+-  SaturateOnIntegerOverflow=on  InputSameDT=on  OutDataTypeStr=Inherit: Same as first input
  Switch : Switch  Criteria=u2 ~= 0  ZeroCross=off  InputSameDT=on
  Switch1 : Switch  Criteria=u2 ~= 0  ZeroCross=off  InputSameDT=on
  Terminator : Terminator
  Unit Delay : UnitDelay  SampleTime=-1
      settings: AttributesFormatString=InitialValue=%<InitialCondition>
  FM_xxx_fault_rec : Outport  OutDataTypeStr=boolean
  wires:
  df/1 -> Switch1/2
  enRecy/1 -> Logical Operator/2
  dec/1 -> Subtract/2
  inc/1 -> Add/2
  frz/1 -> Switch/2
  S-R Flip-Flop/1 -> FM_xxx_fault_rec/1
  Unit Delay/1 -> Switch/1, Subtract/1, Add/1
  Add/1 -> Switch1/1
  Subtract/1 -> Switch1/3
  Switch1/1 -> Saturation Dynamic/2
  Constant/1 -> Saturation Dynamic/1
  Constant1/1 -> Saturation Dynamic/3
  Saturation Dynamic/1 -> Switch/3
  Constant2/1 -> Relational Operator/1
  Switch/1 -> Relational Operator1/2, Unit Delay/1, Relational Operator/2
  Constant3/1 -> Relational Operator1/1
  Relational Operator1/1 -> Logical Operator/1
  Relational Operator/1 -> S-R Flip-Flop/1
  Logical Operator/1 -> S-R Flip-Flop/2
  S-R Flip-Flop/2 -> Terminator/1

== system sllib/FM_frz/soft ==
  df : Inport  OutDataTypeStr=boolean
  frz : Inport  Port=2  OutDataTypeStr=boolean
  Delay : Delay  DelayLength=1  InitialConditionSource=Input port
      settings: InputPortMap=u0,p4
  Switch : Switch  Criteria=u2 ~= 0  ZeroCross=off  InputSameDT=on
  FM_xxx_fault_soft : Outport
  wires:
  frz/1 -> Switch/2
  Switch/1 -> Delay/1, FM_xxx_fault_soft/1
  df/1 -> Delay/2, Switch/3
  Delay/1 -> Switch/1
